simulink model "LIDAR_Stop"  (R2021a)
settings: Solver=ode1  StartTime=0.0  StopTime=inf  FixedStep=1/30  RelTol=1e-3  EnableMultiTasking=on
undefined symbols (not defined in the file): animation_update_interval, datetime, enable_CG_trace, enable_rearAxle_trace, HIL, plotAxisLimitMode, plotAxisLimits, save_anim_frames, vehicle_length, vehicle_width, X_ic, Y_ic, yaw_ic
libraries: quarc_library x8, simulink x1
settings Model: SimulationMode=external  ExtModeTrigDuration=10000  Creator=Quanser  LastModifiedBy=User
settings SolverCC: AlgebraicLoopSolver=TrustRegion  PositivePriorityOrder=on
settings DataIOCC: ReturnWorkspaceOutputs=off
settings DebuggingCC: PregeneratedLibrarySubsystemCodeDiagnostic=none  SFMachineParentedDataDiag=warning  ArithmeticOperatorsInVariantConditions=warning
settings HardwareCC: ProdBitPerLong=64  ProdLargestAtomicInteger=LongLong  ProdLargestAtomicFloat=Double  ProdLongLongMode=on  ProdHWDeviceType=ARM Compatible->ARM 64-bit (LP64)
settings SFSimCC: CustomCodeUndefinedFunction=UseInterfaceOnly
settings RTWCC: Description=QUARC Linux Nvidia Target (QCar) Using Toolchain  SystemTargetFile=quarc_linux_nvidia.tlc  TemplateMakefile=quarc_default_tmf  Toolchain=QUARC linux_nvidia | gmake (64-bit Windows)  BuildConfiguration=Faster Runs
settings STFCustomTargetCC: TargetLangStandard=C99 (ISO)  ConcurrentExecutionCompliant=on  SystemTargetFile=quarc_linux_nvidia.tlc
settings GRTTargetCC: ParMdlRefBuildCompliant=off  CompOptLevelCompliant=off  CombineOutputUpdateFcns=off  MatFileLogging=off  CPPClassGenCompliant=off  GRTInterface=on  ExtMode=on  ExtModeMexFile=quarc_comm  ExtModeMexArgs='-w -d /tmp -uri %u','tcpip://192.168.2.12:17001'

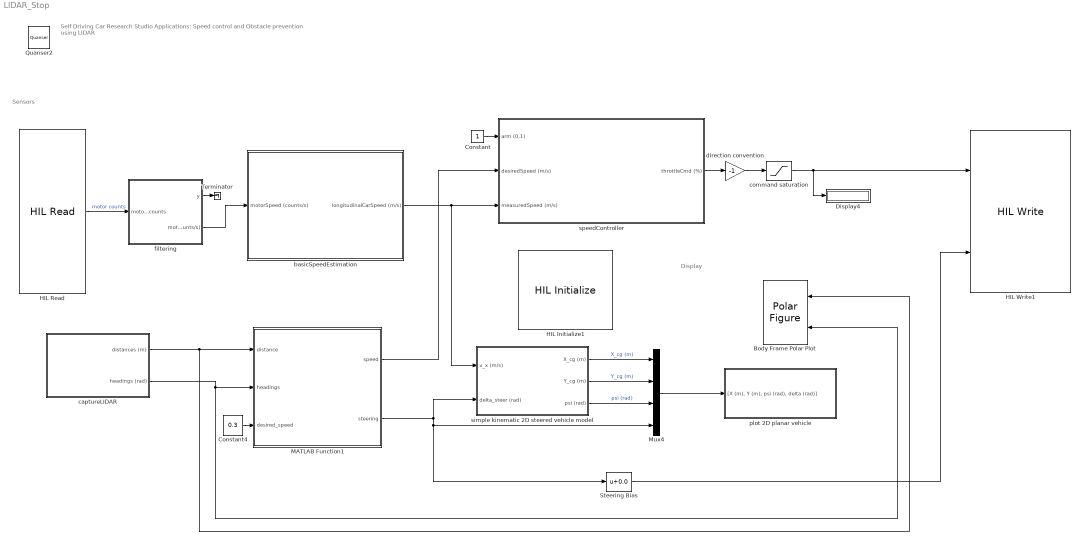
== system LIDAR_Stop ==
  note: Display
  note: Self Driving Car Research Studio
      | Applications: Speed control and Obstacle prevention using LIDAR
  note: Sensors
  Body Frame Polar Plot : quarc_library/Sinks/Figures/Polar Figure  figure_mode=Use figure window  figure_tag=figure1  axes_tag=axes1  plot_mode=Frame-based  minimum_rho=0  maximum_rho=4  minimum_theta=0  maximum_theta=360  zero_location=top  direction=counterclockwise  buffer_size=1000  update_rate=1  sample_time=-1  initial_position="931  -49  958  961"  initial_visibility=off  line1_style=None  line1_width=0.5  line1_color=[0 0.4470 0.7410]  marker1=Circle (o)  marker1_size=1  marker1_edge_color=[0 0.447059 0.741176]  marker1_face_color=[0 0.447059 0.741176]  line2_style=Solid line (-)  line2_width=0.5  line2_color=[0.85098 0.32549 0.0980392]  marker2=None  marker2_size=6  marker2_edge_color=[0.85098 0.32549 0.0980392]  marker2_face_color=[0.85098 0.32549 0.0980392]  line3_style=Solid line (-)  line3_width=0.5  line3_color=[0.929412 0.694118 0.12549]  marker3=None  marker3_size=6  marker3_edge_color=[0.929412 0.694118 0.12549]  marker3_face_color=[0.929412 0.694118 0.12549]  line4_style=Solid line (-)  line4_width=0.5  line4_color=[0.494118 0.184314 0.556863]  marker4=None  marker4_size=6  marker4_edge_color=[0.494118 0.184314 0.556863]  marker4_face_color=[0.494118 0.184314 0.556863]  line5_style=Solid line (-)  line5_width=0.5  line5_color=[0.466667 0.67451 0.188235]  marker5=None  marker5_size=6  marker5_edge_color=[0.466667 0.67451 0.188235]  marker5_face_color=[0.466667 0.67451 0.188235]
      settings: SourceProductName=QUARC Targets
  Constant : Constant
  Constant4 : Constant  Value=0.3
  Display4 : Display
  HIL Initialize1 : quarc_library/Data Acquisition/Generic/Configuration/HIL Initialize  object_name=HIL-1  board_type=qcar  board_number=0  board_options=""  exclusive=off  active=on  hardware_clocks=[]  clock_modes=[]  initial_clock_frequencies=[]  set_clock_params_at_start=off  set_clock_params_at_switch_in=off  set_clock_frequencies_at_start=off  set_clock_frequencies_at_switch_in=off  analog_input_channels=[0:6]  analog_input_configurations=[]  analog_input_maximums=[3.3]  analog_input_minimums=[0]  set_analog_input_params_at_start=off  set_analog_input_params_at_switch_in=off  analog_output_channels=[]  analog_output_maximums=[]  analog_output_minimums=[]  initial_analog_outputs=[]  final_analog_outputs=[]  watchdog_analog_outputs=[]  set_analog_output_params_at_start=off  set_analog_output_params_at_switch_in=off  set_analog_outputs_at_start=off  set_analog_outputs_at_switch_in=off  set_analog_outputs_at_terminate=off  set_analog_outputs_at_switch_out=off  set_analog_outputs_on_watchdog=off  digital_input_channels=[24:42]  digital_output_channels=[40]  digital_output_configuration=[]  initial_digital_outputs=[0]  final_digital_outputs=[1]  watchdog_digital_outputs=[]  set_digital_output_params_at_start=off  set_digital_output_params_at_switch_in=off  set_digital_outputs_at_start=on  set_digital_outputs_at_switch_in=off  set_digital_outputs_at_terminate=on  set_digital_outputs_at_switch_out=off  set_digital_outputs_on_watchdog=off  encoder_channels=[0:4]  quadrature=[4 4]  encoder_filter_frequency=100e6/1  initial_encoder_counts=[0]  set_encoder_params_at_start=on  set_encoder_params_at_switch_in=off  set_encoder_counts_at_start=on  set_encoder_counts_at_switch_in=off  pwm_channels=[0]  pwm_modes=[0 0]  pwm_frequency=150e6/4096  pwm_configuration=[0]  pwm_alignment=[0]  pwm_polarity=[1]  pwm_leading_deadband=[]  pwm_trailing_deadband=[]  initial_pwm_outputs=[0]  final_pwm_outputs=[0]  watchdog_pwm_outputs=[0]  set_pwm_params_at_start=on  set_pwm_params_at_switch_in=off  set_pwm_outputs_at_start=on  set_pwm_outputs_at_switch_in=off  set_pwm_outputs_at_terminate=on  set_pwm_outputs_at_switch_out=off  set_pwm_outputs_on_watchdog=off  other_output_channels=[1000, 11000:11011]  initial_other_outputs=[0]  final_other_outputs=[0]  watchdog_other_outputs=[]  set_other_outputs_at_start=on  set_other_outputs_at_switch_in=off  set_other_outputs_at_terminate=on  set_other_outputs_at_switch_out=off  set_other_outputs_on_watchdog=off
  HIL Read : quarc_library/Data Acquisition/Generic/Immediate I//O/HIL Read  object_name=HIL-1  analog_channels=[]  encoder_channels=[0]  digital_channels=[]  other_channels=[]  sample_time=qc_get_step_size  active=on  vector_output=off  data_type_mode=Inherit via back propagation  encoder_data_type=double  digital_data_type=boolean
  HIL Write1 : quarc_library/Data Acquisition/Generic/Immediate I//O/HIL Write  object_name=HIL-1  analog_channels=[]  pwm_channels=[0]  digital_channels=[]  other_channels=[1000]  sample_time=-1  active=off  vector_input=off
  MATLAB Function1 : MATLAB Function  TreatAsAtomicUnit=on
  Mux4 : Mux
  Quanser2 : quarc_library/Logos/Quanser
  Steering Bias : Bias  Bias=0.0
  Terminator : Terminator
  basicSpeedEstimation : Subsystem
  captureLIDAR : Subsystem
  command saturation : Saturate  UpperLimit=0.20  LowerLimit=-0.20
  direction convention : Gain  Gain=-1
  filtering : Subsystem
  plot 2D planar vehicle : Subsystem  mask(6DoF Animation){axisMode=plotAxisLimitMode, ax=plotAxisLimits, Ts=animation_update_interval, enable_CG_trace=enable_CG_trace, enable_rearAxle_trace=enable_rearAxle_trace, save_anim_frames=save_anim_frames, anim_frame_name_str=char(datetime('now','Format','yyyy-MM-dd_HH_mm_ss')), L=vehicle_length, W=vehicle_width}
      mask prompts: axisMode "Axis Mode (0->auto, 1->fixed, BOTH use Axes Limits below)"; ax "Axes limits [xmin xmax ymin ymax] (m):"; Ts "Time interval between updates (s):"; enable_CG_trace "Enable vehicle CG trace? (0/1)"; enable_rearAxle_trace "Enable rear axle trace? (0/1)"; save_anim_frames "Save animaton frames? (0/1)"; anim_frame_name_str "Animation sequence name (if save frames==1)"; L "Vehicle length (m)"; W "Vehicle width (m)"
      mask help:
      | Create a 2D animated view of a steering vehicle model with tires.
      |
      | Marc Compere
      | CompereM@saic.com
      | created : 22 August 2002
      | modified: 28 Dec 2015
      mask init:
      | Config.axisMode=axisMode;
      | Config.ax=ax;
      | Config.Ts=Ts;
      | Config.enable_CG_trace=enable_CG_trace;
      | Config.enable_rearAxle_trace=enable_rearAxle_trace;
      | Config.save_anim_frames=save_anim_frames;
      | Config.anim_frame_name_str=anim_frame_name_str;
      | Config.L=L;
      | Config.W=W;
      mask Help:
      | <p>This block generates a 3 dimensional display of a simulation trajectory, with the craft orientation displayed during flight</p>
      | 
      | <p>There are two inputs to this block, Position and Euler.  These inputs contain more than one signal as described below.</p>
      | 
      | <p><H4>Block Vector Input - Position</H4>
      | <ul>
      | <li>X Position</li>
      | <li>Y Position</li>
      | <li>Z Position</li>
      | </ul>
      | </p>
      | 
      | <p><H4>Block Vector Input - Euler</H4>
      |     <ul>
      |     <li>Roll Attitude</li>
      |     <li>Pitch Attitude</li>
      |     <li>Yaw Attitude</li>
      |    </ul>
      |    </p>
  simple kinematic 2D steered vehicle model : Subsystem
  speedController : Subsystem
  wires:
  Constant/1 -> speedController/1(arm (0,1))
  basicSpeedEstimation/1(longitudinalCarSpeed (m/s)) -> simple kinematic 2D steered vehicle model/1(v_x (m/s)), speedController/3(measuredSpeed (m/s))
  speedController/1(throttleCmd (%)) -> direction convention/1
  direction convention/1 -> command saturation/1
  command saturation/1 -> Display4/1, HIL Write1/1
  captureLIDAR/1(distances (m)) -> Body Frame Polar Plot/1, MATLAB Function1/1(distance)
  captureLIDAR/2(headings (rad)) -> Body Frame Polar Plot/2, MATLAB Function1/2(headings)
  MATLAB Function1/2(steering) -> Steering Bias/1, Mux4/4, simple kinematic 2D steered vehicle model/2(delta_steer (rad))
  Steering Bias/1 -> HIL Write1/2
  Mux4/1 -> plot 2D planar vehicle/1("[X (m), Y (m), psi (rad), delta (rad)]")
  simple kinematic 2D steered vehicle model/3(psi (rad)) -> Mux4/3  "psi (rad)"
  simple kinematic 2D steered vehicle model/2(Y_cg (m)) -> Mux4/2  "Y_cg (m)"
  simple kinematic 2D steered vehicle model/1(X_cg (m)) -> Mux4/1  "X_cg (m)"
  Constant4/1 -> MATLAB Function1/3(desired_speed)
  MATLAB Function1/1(speed) -> speedController/2(desiredSpeed (m/s))
  HIL Read/1 -> filtering/1(motor counts)  "motor counts"
  filtering/1(y) -> Terminator/1
  filtering/2(motor omega (counts/s)) -> basicSpeedEstimation/1(motorSpeed (counts/s))

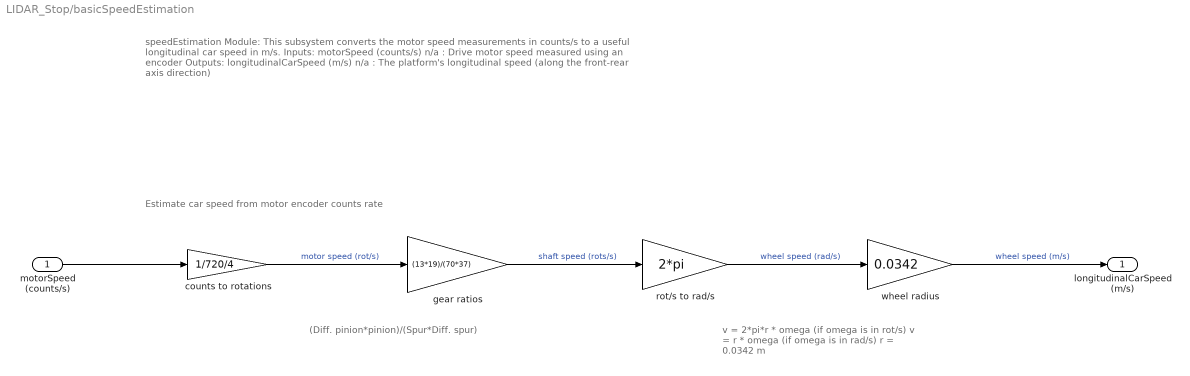
== system LIDAR_Stop/basicSpeedEstimation ==
  note: Estimate car speed from motor encoder counts rate
  note: v = 2*pi*r * omega (if omega is in rot/s)
      | v = r * omega (if omega is in rad/s)
      | r = 0.0342 m
  note: (Diff. pinion*pinion)/(Spur*Diff. spur)
  note: speedEstimation Module:
      |
      | This subsystem converts the motor speed measurements in counts/s to a useful longitudinal car speed in m/s.
      |
      | Inputs:
      | motorSpeed (counts/s) n/a : Drive motor speed measured using an encoder
      |
      | Outputs:
      | longitudinalCarSpeed (m/s) n/a : The platform's longitudinal speed (along the front-rear axis direction)
  motorSpeed (counts/s) : Inport
  counts to rotations : Gain  Gain=1/720/4
  gear ratios : Gain  Gain=(13*19)/(70*37)
  rot/s to rad/s : Gain  Gain=2*pi
  wheel radius : Gain  Gain=0.0342
  longitudinalCarSpeed (m/s) : Outport  VectorParamsAs1DForOutWhenUnconnected=off
  wires:
  motorSpeed (counts/s)/1 -> counts to rotations/1
  rot/s to rad/s/1 -> wheel radius/1  "wheel speed (rad/s)"
  counts to rotations/1 -> gear ratios/1  "motor speed (rot/s)"
  wheel radius/1 -> longitudinalCarSpeed (m/s)/1  "wheel speed (m/s)"
  gear ratios/1 -> rot/s to rad/s/1  "shaft speed (rots/s)"

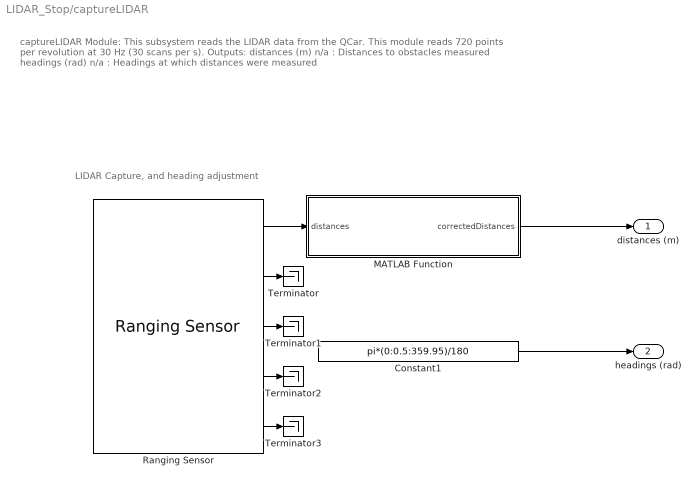
== system LIDAR_Stop/captureLIDAR ==
  note: LIDAR Capture, and heading adjustment
  note: captureLIDAR Module:
      |
      | This subsystem reads the LIDAR data from the QCar. This module reads 720 points per revolution at 30 Hz (30 scans per s).
      |
      | Outputs:
      | distances (m) n/a : Distances to obstacles measured
      | headings (rad) n/a : Headings at which distances were measured
  Constant1 : Constant  Value=pi*(0:0.5:359.95)/180
  MATLAB Function : MATLAB Function  TreatAsAtomicUnit=on
  Ranging Sensor : quarc_library/Devices/Third-Party/Sensors/Ranging Sensor  sensor_type=RPLidar LIDAR  uri=serial-cpu://localhost:2?baud='115200',word='8',parity='none',stop='1',flow='none',dsr='on'  ranging_distance=Long  timing_budget=0.033  measurement_period=0.0001  output_mode=Fixed-size interpolated output  samples_per_revolution=720  max_distance=Inf  max_angle=5  sample_time=qc_get_step_size  active=on
      settings: SourceProductName=QUARC Targets
  Terminator{,1..3} (4 alike) : Terminator
  distances (m) : Outport  VectorParamsAs1DForOutWhenUnconnected=off
  headings (rad) : Outport  Port=2  VectorParamsAs1DForOutWhenUnconnected=off
  wires:
  Ranging Sensor/1 -> MATLAB Function/1(distances)
  MATLAB Function/1(correctedDistances) -> distances (m)/1
  Constant1/1 -> headings (rad)/1
  Ranging Sensor/2 -> Terminator/1
  Ranging Sensor/3 -> Terminator1/1
  Ranging Sensor/4 -> Terminator2/1
  Ranging Sensor/5 -> Terminator3/1

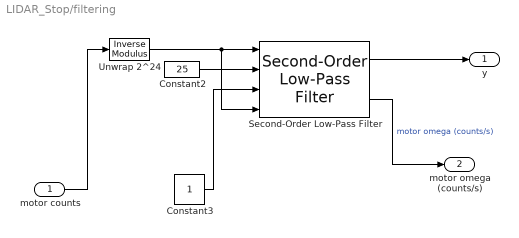
== system LIDAR_Stop/filtering ==
  motor counts : Inport
  Constant2 : Constant  Value=25
  Constant3 : Constant
  Second-Order Low-Pass Filter : quarc_library/Continuous/Second-Order Low-Pass Filter  params_source=External (input ports)  input_width=1  input_zeta=1  input_init=0
  Unwrap 2^24 : quarc_library/Discontinuities/Inverse Modulus  modulus=16777215  output_derivative=off  output_revolutions=off  max_x=Inf  min_x=-Inf
  y : Outport
  motor omega (counts/s) : Outport  Port=2
  wires:
  Unwrap 2^24/1 -> Second-Order Low-Pass Filter/4, Second-Order Low-Pass Filter/1
  Second-Order Low-Pass Filter/1 -> y/1
  Constant3/1 -> Second-Order Low-Pass Filter/3
  Second-Order Low-Pass Filter/2 -> motor omega (counts/s)/1  "motor omega (counts/s)"
  Constant2/1 -> Second-Order Low-Pass Filter/2
  motor counts/1 -> Unwrap 2^24/1

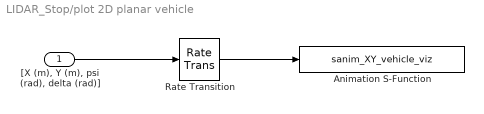
== system LIDAR_Stop/plot 2D planar vehicle ==
  "[X (m), Y (m), psi (rad), delta (rad)]" : Inport
  Animation S-Function : S-Function  FunctionName=sanim_XY_vehicle_viz  Parameters=Config  SFunctionDeploymentMode=off  EnableBusSupport=off
  Rate Transition : RateTransition  Integrity=off
  wires:
  "[X (m), Y (m), psi (rad), delta (rad)]"/1 -> Rate Transition/1
  Rate Transition/1 -> Animation S-Function/1

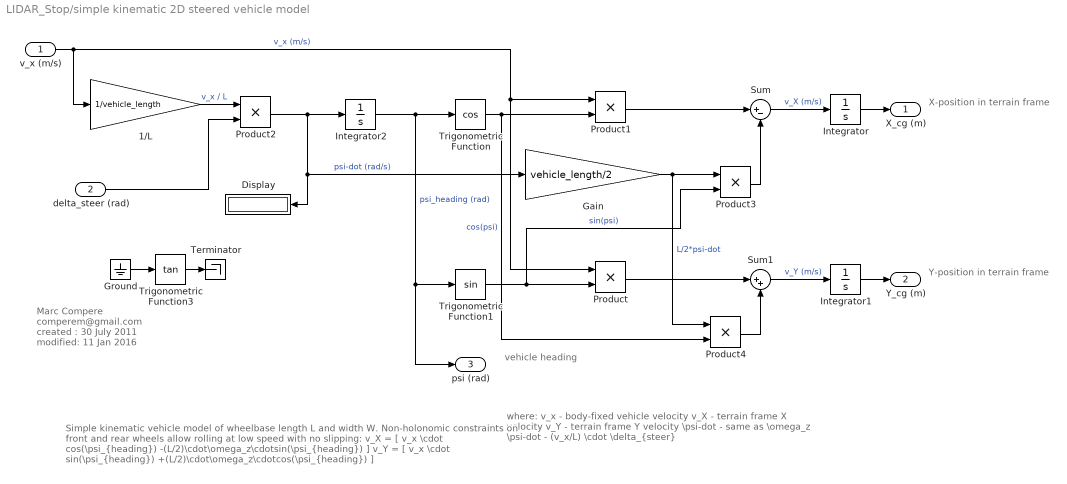
== system LIDAR_Stop/simple kinematic 2D steered vehicle model ==
  note: where:
      |    v_x - body-fixed vehicle velocity
      |    v_X - terrain frame X velocity
      |    v_Y - terrain frame Y velocity
      |    \psi-dot - same as \omega_z
      |    \psi-dot - (v_x/L) \cdot \delta_{steer}
  note: X-position in
      | terrain frame
  note: Simple kinematic vehicle model of wheelbase
      | length L and width W.
      | Non-holonomic constraints on front and rear wheels
      | allow rolling at low speed with no slipping:
      |
      |    v_X = [ v_x \cdot cos(\psi_{heading}) -(L/2)\cdot\omega_z\cdotsin(\psi_{heading}) ]
      |    v_Y = [ v_x \cdot sin(\psi_{heading}) +(L/2)\cdot\omega_z\cdotcos(\psi_{heading}) ]
  note: vehicle
      | heading
  note: Marc Compere
      | comperem@gmail.com
      | created : 30 July 2011
      | modified: 11 Jan 2016
  note: Y-position in
      | terrain frame
  v_x (m/s) : Inport
  delta_steer (rad) : Inport  Port=2
  1/L : Gain  Gain=1/vehicle_length
  Display : Display
  Gain : Gain  Gain=vehicle_length/2
  Ground : Ground
  Integrator : Integrator  InitialCondition=X_ic
  Integrator1 : Integrator  InitialCondition=Y_ic
  Integrator2 : Integrator  InitialCondition=yaw_ic
  Product{,1..4} (5 alike) : Product  RndMeth=Zero
  Sum : Sum  Inputs=|+-
  Sum1 : Sum  Inputs=|++
  Terminator : Terminator
  Trigonometric Function : Trigonometry  Operator=cos
  Trigonometric Function1 : Trigonometry
  Trigonometric Function3 : Trigonometry  Operator=tan
  X_cg (m) : Outport  VectorParamsAs1DForOutWhenUnconnected=off
  Y_cg (m) : Outport  Port=2  VectorParamsAs1DForOutWhenUnconnected=off
  psi (rad) : Outport  Port=3  VectorParamsAs1DForOutWhenUnconnected=off
  wires:
  Product/1 -> Sum1/1
  Product1/1 -> Sum/1
  Trigonometric Function/1 -> Product4/2, Product1/2  "cos(psi)"
  Trigonometric Function1/1 -> Product/2, Product3/2  "sin(psi)"
  Integrator2/1 -> Trigonometric Function/1, Trigonometric Function1/1, psi (rad)/1  "psi_heading (rad)"
  Integrator/1 -> X_cg (m)/1
  Integrator1/1 -> Y_cg (m)/1
  v_x (m/s)/1 -> Product/1, Product1/1, 1/L/1  "v_x (m/s)"
  Product2/1 -> Gain/1, Display/1, Integrator2/1  "psi-dot (rad/s)"
  1/L/1 -> Product2/1  "v_x / L"
  Sum/1 -> Integrator/1  "v_X (m/s)"
  Sum1/1 -> Integrator1/1  "v_Y (m/s)"
  Gain/1 -> Product4/1, Product3/1  "L/2*psi-dot"
  Product3/1 -> Sum/2
  Product4/1 -> Sum1/2
  delta_steer (rad)/1 -> Product2/2
  Ground/1 -> Trigonometric Function3/1
  Trigonometric Function3/1 -> Terminator/1

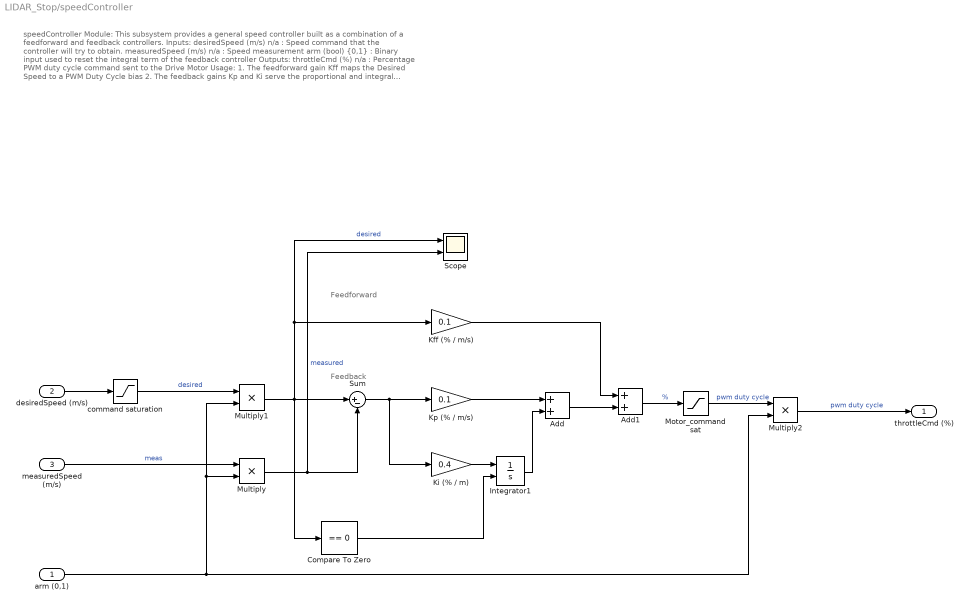
== system LIDAR_Stop/speedController ==
  note: speedController Module:
      |
      | This subsystem provides a general speed controller built as a combination of a feedforward and feedback controllers.
      |
      | Inputs:
      | desiredSpeed (m/s) n/a : Speed command that the controller will try to obtain.
      | measuredSpeed (m/s) n/a : Speed measurement
      | arm (bool) {0,1} : Binary input used to reset the integral term of the feedback controller
      |
      | Outputs:
      | throttleCmd (%) n/a : Percentage PWM duty cycle command sent to the Drive Motor
      |
      | Usage:
      | 1. The feedforward gain Kff maps the Desired Speed to a PWM Duty Cycle bias
      | 2. The feedback gains Kp and Ki serve the proportional and integral terms to output corrections to the PWM Duty Cycle so as to regulate the desired speed.
  note: Feedback
  note: Feedforward
  arm (0,1) : Inport
  desiredSpeed (m/s) : Inport  Port=2
  measuredSpeed (m/s) : Inport  Port=3
  Add : Sum
  Add1 : Sum
  Compare To Zero : simulink/Logic and Bit Operations/Compare To Zero  relop===  OutDataTypeStr=boolean
  Integrator1 : Integrator  ExternalReset=either  LimitOutput=on  UpperSaturationLimit=0.1  LowerSaturationLimit=-0.1
  Kff (% / m/s) : Gain  Gain=0.1
  "Ki (% / m) " : Gain  Gain=0.4
  Kp (% / m/s) : Gain  Gain=0.1
  Motor_command sat : Saturate  LinearizeAsGain=off
  Multiply : Product
  Multiply1 : Product
  Multiply2 : Product
  Scope : Scope  NumInputPorts=2
  Sum : Sum  Inputs=|+-
  command saturation : Saturate  UpperLimit=0.8  LowerLimit=-0.8
  throttleCmd (%) : Outport  VectorParamsAs1DForOutWhenUnconnected=off
  wires:
  desiredSpeed (m/s)/1 -> command saturation/1
  "Ki (% / m) "/1 -> Integrator1/1
  Sum/1 -> Kp (% / m/s)/1, "Ki (% / m) "/1
  Kff (% / m/s)/1 -> Add1/1
  Compare To Zero/1 -> Integrator1/2
  Kp (% / m/s)/1 -> Add/1
  Multiply2/1 -> throttleCmd (%)/1  "pwm duty cycle"
  Integrator1/1 -> Add/2
  Multiply1/1 -> Scope/1, Kff (% / m/s)/1, Sum/1, Compare To Zero/1  "desired"
  Add1/1 -> Motor_command sat/1  "%"
  Motor_command sat/1 -> Multiply2/1  "pwm duty cycle"
  Add/1 -> Add1/2
  Multiply/1 -> Scope/2, Sum/2  "measured"
  measuredSpeed (m/s)/1 -> Multiply/1  "meas"
  arm (0,1)/1 -> Multiply2/2, Multiply/2, Multiply1/2
  command saturation/1 -> Multiply1/1  "desired"

== matlab function LIDAR_Stop/MATLAB Function1 ==
  data: distance input; speed output; headings input; desired_speed input; steering output
function [speed , steering]  = stop(distance, headings,desired_speed)
    X = headings == 0*pi/180;
    
    X1 = headings <= 30*pi/180;
    X2 = headings >= 330*pi/180;
    
    Y1 = distance <= 1 & distance >= 0.1;
    
    calc1 = X1.*Y1;
    calc4 = X2.*Y1;
    
    if max(calc1) == 1 && max(calc4) == 1 %  in the cone, atleast one point is present in point cloud map
        speed = 0;
        steering = 0;    
    else
        speed = desired_speed;
        steering = 0;
    end

== matlab function LIDAR_Stop/captureLIDAR/MATLAB Function ==
  data: distances input; correctedDistances output
function correctedDistances = bodyFrameAdjustmentOnCapture(distances)
num = 720;
correctedDistances = [distances(num/4:-1:1,1); distances(num:-1:num/4 + 1,1)];
